simulink model "sfcndemo_cplx"  (Simulink 6.0)
settings: Solver=FixedStepDiscrete  StartTime=0.0  StopTime=10.0  RelTol=1e-3
settings Model: Creator=The MathWorks Inc.  LastModifiedBy=batserve  ExtModeAutoUpdateStatusClock=off
settings DataIOCC: SaveOutput=off  OutputSaveName=y1,y2,y3,y4
settings OptimizationCC: BlockReduction=off  BooleanDataType=off
settings DebuggingCC: CheckExecutionContextPreStartOutputMsg=on  CheckExecutionContextRuntimeOutputMsg=on  SolverPrmCheckMsg=none
settings HardwareCC: TargetUnknown=on

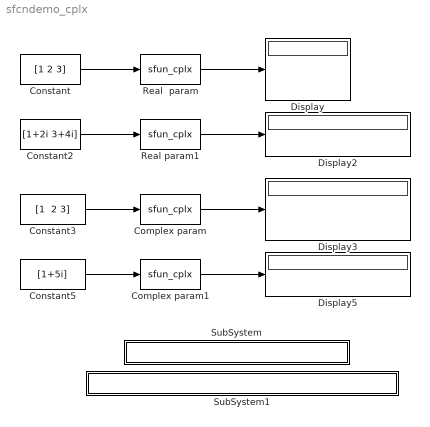
== system sfcndemo_cplx ==
  Complex param : S-Function  FunctionName=sfun_cplx  Parameters=[2+3i 4+5i 6+7i]
      settings: AttributesFormatString=Param = %<Parameters>
  Complex param1 : S-Function  FunctionName=sfun_cplx  Parameters=[1+3i 7+2i]
      settings: AttributesFormatString=Param = %<Parameters>
  Constant : Constant  Value=[1 2 3]  VectorParams1D=off
  Constant2 : Constant  Value=[1+2i 3+4i]  VectorParams1D=off
  Constant3 : Constant  Value="[1  2 3]"  VectorParams1D=off
  Constant5 : Constant  Value=[1+5i]  VectorParams1D=off
  Display{,2..3,5} (4 alike) : Display
  Real  param : S-Function  FunctionName=sfun_cplx  Parameters=5
      settings: AttributesFormatString=Param = %<Parameters>
  Real param1 : S-Function  FunctionName=sfun_cplx  Parameters=[5 6]
      settings: AttributesFormatString=Param = %<Parameters>
  SubSystem : Subsystem  PropExecContextAcrossSSBoundary=on
      settings: OpenFcn=edit(fullfile(matlabroot,'simulink','src','sfun_cplx.c'))
      mask Display: disp('matlabroot\simulink\src\sfun_cplx.c');
  SubSystem1 : Subsystem  PropExecContextAcrossSSBoundary=on
      settings: OpenFcn=edit(fullfile(matlabroot,'toolbox','simulink','blocks','tlc_c','sfun_cplx.tlc'))
      mask Display: disp('matlabroot\toolbox\simulink\blocks\tlc_c\sfun_cplx.tlc');
  wires:
  Constant/1 -> Real  param/1
  Real  param/1 -> Display/1
  Constant2/1 -> Real param1/1
  Real param1/1 -> Display2/1
  Constant3/1 -> Complex param/1
  Complex param/1 -> Display3/1
  Constant5/1 -> Complex param1/1
  Complex param1/1 -> Display5/1

== system sfcndemo_cplx/SubSystem ==

== system sfcndemo_cplx/SubSystem1 ==
